simulink model "ahora_si_perro"  (R2023a)
settings: Solver=VariableStepAuto  StartTime=0.0  StopTime=200000  RelTol=1e-3
settings Model: Creator=Nacho Andrade  LastModifiedBy=Nacho Andrade

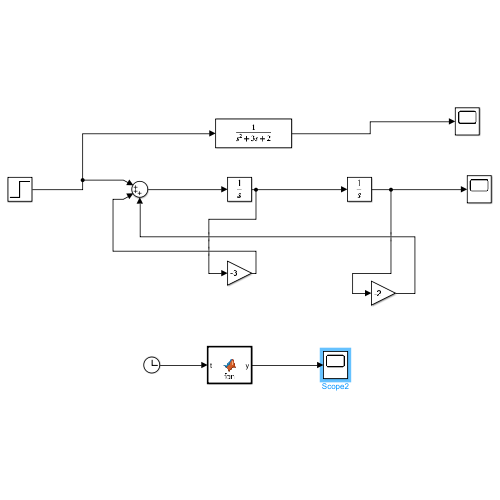
[thumbnail: Simulink's stored preview of the top-level diagram]
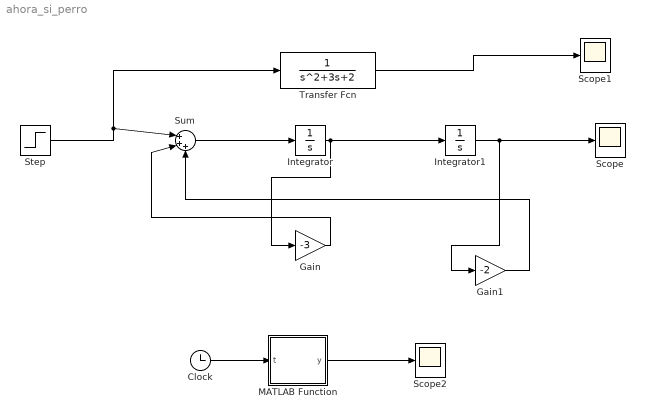
== system ahora_si_perro ==
  Clock : Clock
  Gain : Gain  Gain=-3
  Gain1 : Gain  Gain=-2
  Integrator : Integrator
  Integrator1 : Integrator
  MATLAB Function : MATLAB Function  TreatAsAtomicUnit=on
  Scope : Scope
  Scope1 : Scope
  Scope2 : Scope
  Step : Step  Before=1  After=3  SampleTime=0
  Sum : Sum  Inputs=|+++
  Transfer Fcn : TransferFcn  Denominator=[1 3 2]
  wires:
  Integrator/1 -> Gain/1, Integrator1/1
  Sum/1 -> Integrator/1
  Step/1 -> Transfer Fcn/1, Sum/1
  Integrator1/1 -> Scope/1, Gain1/1
  Gain/1 -> Sum/2
  Gain1/1 -> Sum/3
  Transfer Fcn/1 -> Scope1/1
  Clock/1 -> MATLAB Function/1(t)
  MATLAB Function/1(y) -> Scope2/1

== matlab function ahora_si_perro/MATLAB Function ==
  data: t input; y output
function y = fcn(t)

y = 12*(1-exp(-1/(231.48*240)*t));
